simulink model "CompletePhysicalTireSystem"  (R2025b)
settings: Solver=FixedStepAuto  StartTime=0.0  StopTime=150  FixedStep=0.001  RelTol=1e-3
undefined symbols (not defined in the file): const_mode, init_pressure
libraries: fl_lib x8, nesl_utility x7, SimscapeFluids_lib x3, simulink x1, slpidlib x1
(part 1 of 3)
settings Model: Creator=kimsv  LastModifiedBy=kimsv

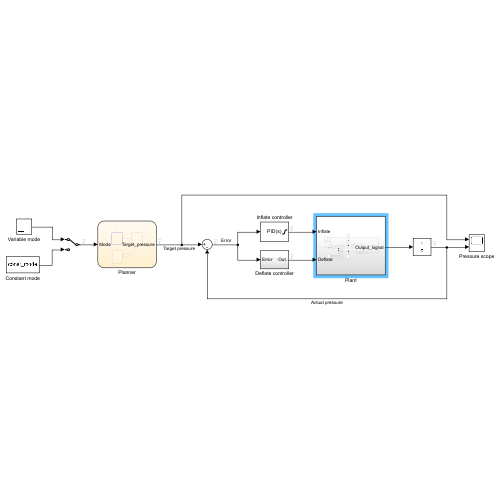
[thumbnail: Simulink's stored preview of the top-level diagram]
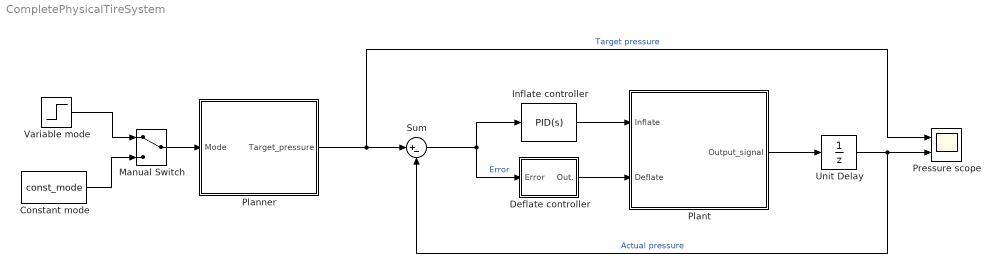
== system CompletePhysicalTireSystem ==
  Constant mode : Constant  Value=const_mode
  Deflate controller : Subsystem
  Inflate controller : slpidlib/PID Controller  Controller=PID  Form=Parallel  TimeDomain=Continuous-time  UseExternalTs=off  SampleTime=-1  IntegratorMethod=Forward Euler  FilterMethod=Forward Euler  ControllerParametersSource=internal  P=0.0105360272273706  I=0.000505771564060444  UseKiTs=off  D=0  UseExternalDerivativeSource=off  N=100  UseFilter=on  TunerSelectOption=Transfer Function Based (PID Tuner App)  InitialConditionSource=internal  InitialConditionForIntegrator=0  InitialConditionForFilter=0  DifferentiatorICPrevScaledInput=0  ExternalReset=none  TrackingMode=off  Kt=1  LimitOutput=on  SatLimitsSource=internal  UpperSaturationLimit=0.0029  LowerSaturationLimit=0  LinearizeAsGain=on  AntiWindupMode=back-calculation  Kb=1  LimitIntegrator=off  UpperIntegratorSaturationLimit=inf  LowerIntegratorSaturationLimit=-inf  POutMin=[]  POutMax=[]  IOutMin=[]  IOutMax=[]  DOutMin=[]  DOutMax=[]  NOutMin=[]  NOutMax=[]  SumOutMin=[]  SumOutMax=[]  SaturationOutMin=[]  SaturationOutMax=[]  PParamMin=[]  PParamMax=[]  IParamMin=[]  IParamMax=[]  DParamMin=[]  DParamMax=[]  NParamMin=[]  NParamMax=[]  KbParamMin=[]  KbParamMax=[]  KtParamMin=[]  KtParamMax=[]  KbOutMin=[]  KbOutMax=[]  KtOutMin=[]  KtOutMax=[]  IntegratorOutMin=[]  IntegratorOutMax=[]  FilterOutMin=[]  FilterOutMax=[]  SumI1OutMin=[]  SumI1OutMax=[]  SumI2OutMin=[]  SumI2OutMax=[]  SumI3OutMin=[]  SumI3OutMax=[]  SumI4OutMin=[]  SumI4OutMax=[]  SumDOutMin=[]  SumDOutMax=[]  DifferentiatorOutMin=[]  DifferentiatorOutMax=[]  FilterDiffOutCoefMin=[]  FilterDiffOutCoefMax=[]  ReciprocalOutMin=[]  ReciprocalOutMax=[]  SumDenOutMin=[]  SumDenOutMax=[]  SumNumOutMin=[]  SumNumOutMax=[]  DivideOutMin=[]  DivideOutMax=[]  UdiffTsProdOutMin=[]  UdiffTsProdOutMax=[]  NTsProdOutMin=[]  NTsProdOutMax=[]  UintegralTsProdOutMin=[]  UintegralTsProdOutMax=[]  UngainTsProdOutMin=[]  UngainTsProdOutMax=[]  ClampingZeroOutDataTypeStr=Inherit: Inherit via back propagation  ClampingZeroOutMin=[]  ClampingZeroOutMax=[]  FilterDenConstantOutDataTypeStr=Inherit: Inherit via back propagation  FilterDenConstantOutMin=[]  FilterDenConstantOutMax=[]  PCopyOutDataTypeStr=Inherit: Inherit via back propagation  PCopyOutMin=[]  PCopyOutMax=[]  NCopyOutDataTypeStr=Inherit: Inherit via back propagation  NCopyOutMin=[]  NCopyOutMax=[]  IntegratorContinuousStateAttributes=''  IntegratorStateMustResolveToSignalObject=off  IntegratorRTWStateStorageClass=Auto  FilterContinuousStateAttributes=''  FilterStateMustResolveToSignalObject=off  FilterRTWStateStorageClass=Auto  ParallelPVariant=InternalParameters  IdealPVariant=Disabled  IVariant=InternalParameters  DVariant=InternalParameters  IntegratorVariant=Continuous  SatVariant=Enabled  AWVariant=BackCalculation  PCopyVariant=Disabled  TRVariant=Disabled  FdbkBlocksVariant=Forward  IdealPFdbkVariant=Disabled  SatFdbkVariant=Disabled  DerivativeFilterVariant=ContFilter  NVariant=InternalParameters  NCopyVariant=Disabled  FilterICVariant=InternalICsFilter  IntegratorICVariant=InternalICs  ExternalResetVariant=Disabled  TRSumVariant=Passthrough  SumFdbkVariant=Disabled  SumVariant=Sum_PID  TsampFilterVariant=InternalTs  TsampNgainVariant=Passthrough  TsampIntegralVariant=Disabled_SignalSpec  ExternalSaturationOutDataTypeStr=Inherit: Same as second input  DerivativeSourceVariant=ErrorSignal  PreIntVariant=InternalPreInt
  Manual Switch : ManualSwitch
  Planner : Stateflow chart  TreatAsAtomicUnit=on
  Plant : Subsystem
  Pressure scope : Scope  NumInputPorts=2
      settings: ActiveDisplayYMinimum=0.78749999999999987  ActiveDisplayYMaximum=2.9125
  Sum : Sum  Inputs=|+-
  Unit Delay : UnitDelay  InitialCondition=init_pressure  SampleTime=0.01  HasFrameUpgradeWarning=on
  Variable mode : Step  Time=100  SampleTime=0
  wires:
  Planner/1(Target_pressure) -> Sum/1, Pressure scope/1  "Target pressure"
  Inflate controller/1 -> Plant/1(Inflate)
  Sum/1 -> Deflate controller/1(Error), Inflate controller/1  "Error"
  Plant/1(Output_signal) -> Unit Delay/1
  Unit Delay/1 -> Pressure scope/2, Sum/2  "Actual pressure"
  Constant mode/1 -> Manual Switch/2
  Variable mode/1 -> Manual Switch/1
  Manual Switch/1 -> Planner/1(Mode)
  Deflate controller/1(Out.) -> Plant/2(Deflate)

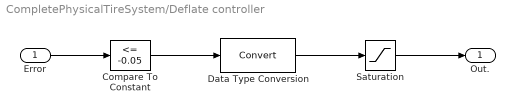
== system CompletePhysicalTireSystem/Deflate controller ==
  Error : Inport
  Compare To Constant : simulink/Logic and Bit Operations/Compare To Constant  relop=<=  const=-0.05  OutDataTypeStr=boolean
  Data Type Conversion : DataTypeConversion  SaturateOnIntegerOverflow=off  RndMeth=Floor
  Saturation : Saturate  UpperLimit=0.15  LowerLimit=0
  Out. : Outport
  wires:
  Error/1 -> Compare To Constant/1
  Saturation/1 -> Out./1
  Compare To Constant/1 -> Data Type Conversion/1
  Data Type Conversion/1 -> Saturation/1
